simulink model "SIMULINK_FT_SRL_NZS_Tracking_R18b"  (R2018b)
settings: Solver=FixedStepAuto  StartTime=0.0  StopTime=sim_end_time  FixedStep=fixed_step_size  RelTol=1e-3
InitFcn:
  | start_uav_car_10
values from neighbouring files (symbols this model uses):
  a = 1    [start_uav_car_10.m]
  act_end = 2*pi/w1    (= 62.8318530718)    [start_uav_car_10.m]
  b = 1.8    [start_uav_car_10.m]
  battery_threshold = 20    [start_uav_car_10.m]
  bb = 1.2    [start_uav_car_10.m]
  delta_ = [delta_his(2:end,:); delta]    [adp_tracking.m]    (also in start_uav_car_10.m = zeros(N,1))
  draw_gif = false    [start_uav_car_10.m]
  fixed_step_size = 1/30    (= 0.0333333333333)    [start_uav_car_10.m]
  k = 0.2    [start_uav_car_10.m]
  KD_x = 0.000002    (= 2e-06)    [start_uav_car_10.m]
  KD_y = 0.00002    (= 2e-05)    [start_uav_car_10.m]
  kd_z = 0.02    [start_uav_car_10.m]
  KDD_x = 0.0008    [start_uav_car_10.m]
  KDD_y = 0.0008    [start_uav_car_10.m]
  KI_x = 0.000002    (= 2e-06)    [start_uav_car_10.m]
  KI_y = 0.000002    (= 2e-06)    [start_uav_car_10.m]
  ki_z = 0.002    [start_uav_car_10.m]
  KII_x = 0.000000    (= 0)    [start_uav_car_10.m]
  KII_y = 0.000    (= 0)    [start_uav_car_10.m]
  KP_x = 1.5    [start_uav_car_10.m]
  KP_y = 1.5    [start_uav_car_10.m]
  kp_z = 0.7    [start_uav_car_10.m]
  KPP_x = 0.4    [start_uav_car_10.m]
  KPP_y = 0.4    [start_uav_car_10.m]
  lmt = 0.5    [start_uav_car_10.m]
  omega = omega_(i,:)    [adp_tracking.m]    (also in start_uav_car_10.m = 0.3)
  omega_ = [omega_his(2:end,:); omega']    [adp_tracking.m]    (also in start_uav_car_10.m = zeros(N,l))
  R = 200*eye(2)    [adp_tracking.m]    (also in start_uav_car_10.m = 0.7)
  sim_end_time = 300    [start_uav_car_10.m]    (also in trjcar.m = 600)
  UAV_NUM = 1    [start_uav_car_10.m]
  Vel_Switch_1 = 1    [start_uav_car_10.m]
  Vel_Switch_10 = 1    [start_uav_car_10.m]
  Vel_Switch_11 = 1    [start_uav_car_10.m]
  Vel_Switch_12 = 1    [start_uav_car_10.m]
  Vel_Switch_13 = 1    [start_uav_car_10.m]
  Vel_Switch_14 = 1    [start_uav_car_10.m]
  Vel_Switch_15 = 1    [start_uav_car_10.m]
  Vel_Switch_16 = 1    [start_uav_car_10.m]
  Vel_Switch_17 = 1    [start_uav_car_10.m]
  Vel_Switch_18 = 1    [start_uav_car_10.m]
  Vel_Switch_19 = 1    [start_uav_car_10.m]
  Vel_Switch_2 = 1    [start_uav_car_10.m]
  Vel_Switch_20 = 1    [start_uav_car_10.m]
  Vel_Switch_3 = 1    [start_uav_car_10.m]
  Vel_Switch_4 = 1    [start_uav_car_10.m]
  Vel_Switch_5 = 1    [start_uav_car_10.m]
  Vel_Switch_6 = 1    [start_uav_car_10.m]
  Vel_Switch_7 = 1    [start_uav_car_10.m]
  Vel_Switch_8 = 1    [start_uav_car_10.m]
  Vel_Switch_9 = 1    [start_uav_car_10.m]
  W0 = 10*ones(l,1)    [start_uav_car_10.m]
  w1 = 0.1    [start_uav_car_10.m]
  w2 = 30    [start_uav_car_10.m]
  XMAX = 2.8    [start_uav_car_10.m]
  XMIN = -2.8    [start_uav_car_10.m]
  YMAX = 2.2    [start_uav_car_10.m]
  YMIN = -2.2    [start_uav_car_10.m]
  ys = ys_learned - ys_learned(1,:)    [start_uav_car_10.m]
  ys_learned = [-20 -19.9842645881 -19.9722755737 -19.9635643089 -19.9577075469 -19.9543235714 -19.9530686431 -19.9536337356 -19.9557415391 -19.9591437091 -19.9636183405 -19.9689676484 ... (12618 elements, 6309x2)]    [DMP_ref.mat]
  z_d_for_land = 1    [start_uav_car_10.m]
  ZMAX = 2.0    (= 2)    [start_uav_car_10.m]
  ZMIN = 0.7    [start_uav_car_10.m]
undefined symbols (not defined in the file or in its folder): droneyeeUAV2_NUM, droneyeeUAV3_NUM, droneyeeUAV4_NUM, droneyeeUAV5_NUM, uav10num, uav1num, uav2num, uav3num, uav4num, uav5num, uav6num, uav7num, uav8num, uav9num
libraries: simulink x121, aerolibanimutils x1
(part 5 of 11)

== system SIMULINK_FT_SRL_NZS_Tracking_R18b/CMD_car1/CMD6 ==
  "clock " : Inport
  droneyeeUAV_states : Inport  Port=2
  droneyeeUAV_bat : Inport  Port=3
  Bus Selector : BusSelector  OutputSignals=x,y,z
  Constant : Constant  Value=sim_end_time
  Constant1 : Constant  Value=battery_threshold
  Constant2 : Constant  Value=z_d_for_land
  Constant3 : Constant  Value=0
  Constant4 : Constant  Value=UAV_NUM
  MATLAB Function1 : MATLAB Function  TreatAsAtomicUnit=on
  Manual Switch2 : ManualSwitch
  Sine Wave2 : Sin  Amplitude=0.3  Frequency=1.0
  Slider Gain3 : simulink/Math Operations/Slider Gain  gain=1  low=0  high=2
  Subsystem : Subsystem
  x_d : Outport
  y_d : Outport  Port=2
  z_d : Outport  Port=3
  yaw_d : Outport  Port=4
  wires:
  Manual Switch2/1 -> Slider Gain3/1
  Slider Gain3/1 -> yaw_d/1
  Sine Wave2/1 -> Manual Switch2/2
  Constant3/1 -> Manual Switch2/1
  MATLAB Function1/2(y_d_) -> y_d/1
  Constant2/1 -> MATLAB Function1/11(z_d_for_land)
  Subsystem/3(zd) -> MATLAB Function1/3(z_d)
  Constant1/1 -> MATLAB Function1/10(battery_threshold)
  MATLAB Function1/3(z_d_) -> z_d/1
  droneyeeUAV_states/1 -> Subsystem/2(uavstates), Bus Selector/1
  MATLAB Function1/1(x_d_) -> x_d/1
  Constant4/1 -> MATLAB Function1/12(UAV_NUM)
  Constant/1 -> MATLAB Function1/9(sim_time_end)
  Subsystem/1("xd ") -> MATLAB Function1/1(x_d)
  Subsystem/2(yd) -> MATLAB Function1/2(y_d)
  "clock "/1 -> Subsystem/1(clock), MATLAB Function1/4(timestamp)
  droneyeeUAV_bat/1 -> MATLAB Function1/8(battery_status)
  Bus Selector/1 -> MATLAB Function1/5(x)  "<x>"
  Bus Selector/2 -> MATLAB Function1/6(y)  "<y>"
  Bus Selector/3 -> MATLAB Function1/7(z)  "<z>"

== system SIMULINK_FT_SRL_NZS_Tracking_R18b/CMD_car1/CMD7 ==
  "clock " : Inport
  droneyeeUAV_states : Inport  Port=2
  droneyeeUAV_bat : Inport  Port=3
  Bus Selector : BusSelector  OutputSignals=x,y,z
  Constant : Constant  Value=sim_end_time
  Constant1 : Constant  Value=battery_threshold
  Constant2 : Constant  Value=z_d_for_land
  Constant3 : Constant  Value=0
  Constant4 : Constant  Value=UAV_NUM
  MATLAB Function1 : MATLAB Function  TreatAsAtomicUnit=on
  Manual Switch2 : ManualSwitch
  Sine Wave2 : Sin  Amplitude=0.3  Frequency=1.0
  Slider Gain3 : simulink/Math Operations/Slider Gain  gain=1  low=0  high=2
  Subsystem : Subsystem
  Terminator : Terminator
  x_d : Outport
  y_d : Outport  Port=2
  z_d : Outport  Port=3
  yaw_d : Outport  Port=4
  wires:
  Manual Switch2/1 -> Slider Gain3/1
  Slider Gain3/1 -> yaw_d/1
  Sine Wave2/1 -> Manual Switch2/2
  Constant3/1 -> Manual Switch2/1
  Bus Selector/1 -> MATLAB Function1/5(x)  "<x>"
  MATLAB Function1/2(y_d_) -> y_d/1
  Constant2/1 -> MATLAB Function1/11(z_d_for_land)
  Subsystem/3(zd) -> MATLAB Function1/3(z_d)
  Bus Selector/2 -> MATLAB Function1/6(y)  "<y>"
  Constant1/1 -> MATLAB Function1/10(battery_threshold)
  MATLAB Function1/3(z_d_) -> z_d/1
  MATLAB Function1/1(x_d_) -> x_d/1
  Constant4/1 -> MATLAB Function1/12(UAV_NUM)
  Bus Selector/3 -> MATLAB Function1/7(z)  "<z>"
  Constant/1 -> MATLAB Function1/9(sim_time_end)
  Subsystem/1("xd ") -> MATLAB Function1/1(x_d)
  Subsystem/2(yd) -> MATLAB Function1/2(y_d)
  "clock "/1 -> Subsystem/1(clock), MATLAB Function1/4(timestamp)
  droneyeeUAV_bat/1 -> MATLAB Function1/8(battery_status)
  droneyeeUAV_states/1 -> Subsystem/2(uavstates), Bus Selector/1

== system SIMULINK_FT_SRL_NZS_Tracking_R18b/CMD_car1/CMD8 ==
  "clock " : Inport
  droneyeeUAV_states : Inport  Port=2
  droneyeeUAV_bat : Inport  Port=3
  Bus Selector : BusSelector  OutputSignals=x,y,z
  Constant : Constant  Value=sim_end_time
  Constant1 : Constant  Value=battery_threshold
  Constant2 : Constant  Value=z_d_for_land
  Constant3 : Constant  Value=0
  Constant4 : Constant  Value=UAV_NUM
  MATLAB Function1 : MATLAB Function  TreatAsAtomicUnit=on
  Manual Switch2 : ManualSwitch
  Sine Wave2 : Sin  Amplitude=0.3  Frequency=1.0
  Slider Gain3 : simulink/Math Operations/Slider Gain  gain=1  low=0  high=2
  Subsystem : Subsystem
  x_d : Outport
  y_d : Outport  Port=2
  z_d : Outport  Port=3
  yaw_d : Outport  Port=4
  wires:
  Manual Switch2/1 -> Slider Gain3/1
  Slider Gain3/1 -> yaw_d/1
  Sine Wave2/1 -> Manual Switch2/2
  Constant3/1 -> Manual Switch2/1
  MATLAB Function1/2(y_d_) -> y_d/1
  Constant2/1 -> MATLAB Function1/11(z_d_for_land)
  Subsystem/3(zd) -> MATLAB Function1/3(z_d)
  Constant1/1 -> MATLAB Function1/10(battery_threshold)
  MATLAB Function1/3(z_d_) -> z_d/1
  droneyeeUAV_states/1 -> Subsystem/2(uavstates), Bus Selector/1
  MATLAB Function1/1(x_d_) -> x_d/1
  Constant4/1 -> MATLAB Function1/12(UAV_NUM)
  Constant/1 -> MATLAB Function1/9(sim_time_end)
  Subsystem/1("xd ") -> MATLAB Function1/1(x_d)
  Subsystem/2(yd) -> MATLAB Function1/2(y_d)
  "clock "/1 -> Subsystem/1(clock), MATLAB Function1/4(timestamp)
  droneyeeUAV_bat/1 -> MATLAB Function1/8(battery_status)
  Bus Selector/1 -> MATLAB Function1/5(x)  "<x>"
  Bus Selector/2 -> MATLAB Function1/6(y)  "<y>"
  Bus Selector/3 -> MATLAB Function1/7(z)  "<z>"

== system SIMULINK_FT_SRL_NZS_Tracking_R18b/CMD_car1/CMD9 ==
  "clock " : Inport
  droneyeeUAV_states : Inport  Port=2
  droneyeeUAV_bat : Inport  Port=3
  Bus Selector : BusSelector  OutputSignals=x,y,z
  Constant : Constant  Value=sim_end_time
  Constant1 : Constant  Value=battery_threshold
  Constant2 : Constant  Value=z_d_for_land
  Constant3 : Constant  Value=0
  Constant4 : Constant  Value=UAV_NUM
  MATLAB Function1 : MATLAB Function  TreatAsAtomicUnit=on
  Manual Switch2 : ManualSwitch
  Sine Wave2 : Sin  Amplitude=0.3  Frequency=1.0
  Slider Gain3 : simulink/Math Operations/Slider Gain  gain=1  low=0  high=2
  Subsystem : Subsystem
  Terminator : Terminator
  x_d : Outport
  y_d : Outport  Port=2
  z_d : Outport  Port=3
  yaw_d : Outport  Port=4
  wires:
  Manual Switch2/1 -> Slider Gain3/1
  Slider Gain3/1 -> yaw_d/1
  Sine Wave2/1 -> Manual Switch2/2
  Constant3/1 -> Manual Switch2/1
  Bus Selector/1 -> MATLAB Function1/5(x)  "<x>"
  MATLAB Function1/2(y_d_) -> y_d/1
  Constant2/1 -> MATLAB Function1/11(z_d_for_land)
  Subsystem/3(zd) -> MATLAB Function1/3(z_d)
  Bus Selector/2 -> MATLAB Function1/6(y)  "<y>"
  Constant1/1 -> MATLAB Function1/10(battery_threshold)
  MATLAB Function1/3(z_d_) -> z_d/1
  MATLAB Function1/1(x_d_) -> x_d/1
  Constant4/1 -> MATLAB Function1/12(UAV_NUM)
  Bus Selector/3 -> MATLAB Function1/7(z)  "<z>"
  Constant/1 -> MATLAB Function1/9(sim_time_end)
  Subsystem/1("xd ") -> MATLAB Function1/1(x_d)
  Subsystem/2(yd) -> MATLAB Function1/2(y_d)
  "clock "/1 -> Subsystem/1(clock), MATLAB Function1/4(timestamp)
  droneyeeUAV_bat/1 -> MATLAB Function1/8(battery_status)
  droneyeeUAV_states/1 -> Subsystem/2(uavstates), Bus Selector/1

== system SIMULINK_FT_SRL_NZS_Tracking_R18b/control system_UAV/Baseline Controller1 ==
  X_e : Inport
  Y_e : Inport  Port=2
  " Z_e " : Inport  Port=3
  Yaw_e : Inport  Port=4
  " V_x" : Inport  Port=5
  V_y : Inport  Port=6
  "V_z " : Inport  Port=7
  x_d : Inport  Port=8
  y_d : Inport  Port=9
  Z_d : Inport  Port=10
  Yaw_d : Inport  Port=11
  Constant : Constant  Commented=on  Value=omega*R*2
  Demux : Demux  Outputs=2
  Heading controller : Subsystem
  "Height controller " : Subsystem
  MATLAB Function : MATLAB Function  Commented=on  TreatAsAtomicUnit=on
  Position controller : Subsystem
  Saturation1 : Saturate  UpperLimit=lmt  LowerLimit=-lmt
  Saturation2 : Saturate  UpperLimit=lmt  LowerLimit=-lmt
  Scope : Scope  NumInputPorts=6
  input : Scope  NumInputPorts=3
  ux : Outport
  uy : Outport  Port=2
  Z_velocity_d. [-1,1] : Outport  Port=3
  yaw_rate_d [-1,1] : Outport  Port=4
  wires:
  " Z_e "/1 -> Scope/5, "Height controller "/2(Z_e (m))  "z"
  X_e/1 -> Scope/1, Position controller/1(X_e (m))  "x"
  Y_e/1 -> Scope/3, Position controller/2(Y_e (m))  "y"
  Yaw_d/1 -> Heading controller/2(yaw_d. (rad))
  Demux/1 -> ux/1
  Demux/2 -> uy/1
  Constant/1 -> MATLAB Function/2(a)
  Z_d/1 -> Scope/6, "Height controller "/1(Z_d. (m))  "zd"
  x_d/1 -> Scope/2, Position controller/3(X_d (m))  "xd"
  y_d/1 -> Scope/4, Position controller/4(Y_d (m))  "yd"
  Yaw_e/1 -> Heading controller/1(yaw_e (rad))  "yaw"
  "V_z "/1 -> "Height controller "/3(V_z)
  "Height controller "/1(Z_velocity_d (m/s)) -> Saturation2/1
  Saturation1/1 -> input/2, Demux/1
  Position controller/1(uxy) -> Saturation1/1
  Saturation2/1 -> input/1, Z_velocity_d. [-1,1]/1
  Heading controller/1(yaw_rate_d. (rad/s)) -> input/3, yaw_rate_d [-1,1]/1

== system SIMULINK_FT_SRL_NZS_Tracking_R18b/control system_UAV/Baseline Controller10 ==
  X_e : Inport
  Y_e : Inport  Port=2
  " Z_e " : Inport  Port=3
  Yaw_e : Inport  Port=4
  " V_x" : Inport  Port=5
  V_y : Inport  Port=6
  "V_z " : Inport  Port=7
  x_d : Inport  Port=8
  y_d : Inport  Port=9
  Z_d : Inport  Port=10
  Yaw_d : Inport  Port=11
  Demux : Demux  Outputs=2
  Heading controller : Subsystem
  "Height controller " : Subsystem
  Position controller : Subsystem
  Saturation : Saturate  UpperLimit=lmt  LowerLimit=-lmt
  Saturation1 : Saturate  UpperLimit=lmt  LowerLimit=-lmt
  Saturation2 : Saturate  UpperLimit=lmt  LowerLimit=-lmt
  Scope : Scope
  ux : Outport
  uy : Outport  Port=2
  Z_velocity_d. [-1,1] : Outport  Port=3
  yaw_rate_d [-1,1] : Outport  Port=4
  wires:
  X_e/1 -> Position controller/1(X_e (m))
  Y_e/1 -> Position controller/2(Y_e (m))
  Yaw_d/1 -> Heading controller/2(yaw_d. (rad))
  Saturation/1 -> Demux/1
  Demux/1 -> Scope/1, ux/1
  Demux/2 -> uy/1
  x_d/1 -> Position controller/3(X_d (m))
  y_d/1 -> Position controller/4(Y_d (m))
  Yaw_e/1 -> Heading controller/1(yaw_e (rad))  "yaw"
  Position controller/1(uxy) -> Saturation/1
  Z_d/1 -> "Height controller "/1(Z_d. (m))
  " Z_e "/1 -> "Height controller "/2(Z_e (m))
  "Height controller "/1(Z_velocity_d (m/s)) -> Saturation2/1
  "V_z "/1 -> "Height controller "/3(V_z)
  Saturation2/1 -> Z_velocity_d. [-1,1]/1

== system SIMULINK_FT_SRL_NZS_Tracking_R18b/control system_UAV/Baseline Controller2 ==
  X_e : Inport
  Y_e : Inport  Port=2
  " Z_e " : Inport  Port=3
  Yaw_e : Inport  Port=4
  " V_x" : Inport  Port=5
  V_y : Inport  Port=6
  "V_z " : Inport  Port=7
  x_d : Inport  Port=8
  y_d : Inport  Port=9
  Z_d : Inport  Port=10
  Yaw_d : Inport  Port=11
  Constant : Constant  Commented=on  Value=omega*R*2
  Demux : Demux  Outputs=2
  Heading controller : Subsystem
  "Height controller " : Subsystem
  MATLAB Function : MATLAB Function  Commented=on  TreatAsAtomicUnit=on
  Position controller : Subsystem
  Saturation : Saturate  UpperLimit=lmt  LowerLimit=-lmt
  Saturation1 : Saturate  UpperLimit=lmt  LowerLimit=-lmt
  ux : Outport
  uy : Outport  Port=2
  Z_velocity_d. [-1,1] : Outport  Port=3
  yaw_rate_d [-1,1] : Outport  Port=4
  wires:
  Position controller/1(uxy) -> Saturation/1
  Yaw_e/1 -> Heading controller/1(yaw_e (rad))  "yaw"
  y_d/1 -> Position controller/4(Y_d (m))
  x_d/1 -> Position controller/3(X_d (m))
  Constant/1 -> MATLAB Function/2(a)
  Demux/2 -> uy/1
  Demux/1 -> ux/1
  Saturation/1 -> Demux/1
  Yaw_d/1 -> Heading controller/2(yaw_d. (rad))
  Y_e/1 -> Position controller/2(Y_e (m))
  X_e/1 -> Position controller/1(X_e (m))
  Z_d/1 -> "Height controller "/1(Z_d. (m))
  " Z_e "/1 -> "Height controller "/2(Z_e (m))
  "V_z "/1 -> "Height controller "/3(V_z)
  Saturation1/1 -> Z_velocity_d. [-1,1]/1
  "Height controller "/1(Z_velocity_d (m/s)) -> Saturation1/1

== system SIMULINK_FT_SRL_NZS_Tracking_R18b/control system_UAV/Baseline Controller3 ==
  X_e : Inport
  Y_e : Inport  Port=2
  " Z_e " : Inport  Port=3
  Yaw_e : Inport  Port=4
  " V_x" : Inport  Port=5
  V_y : Inport  Port=6
  "V_z " : Inport  Port=7
  x_d : Inport  Port=8
  y_d : Inport  Port=9
  Z_d : Inport  Port=10
  Yaw_d : Inport  Port=11
  Add : Sum
  Add1 : Sum
  Constant : Constant  Commented=on  Value=omega*R*2
  Demux : Demux  Outputs=2
  Demux1 : Demux  Outputs=2
  Heading controller : Subsystem
  "Height controller " : Subsystem
  MATLAB Function : MATLAB Function  Commented=on  TreatAsAtomicUnit=on
  Position controller : Subsystem
  Saturation : Saturate  UpperLimit=lmt  LowerLimit=-lmt
  Saturation1 : Saturate  UpperLimit=lmt  LowerLimit=-lmt
  Saturation2 : Saturate  UpperLimit=lmt  LowerLimit=-lmt
  ux : Outport
  uy : Outport  Port=2
  Z_velocity_d. [-1,1] : Outport  Port=3
  yaw_rate_d [-1,1] : Outport  Port=4
  wires:
  X_e/1 -> Position controller/1(X_e (m))
  Y_e/1 -> Position controller/2(Y_e (m))
  Yaw_d/1 -> Heading controller/2(yaw_d. (rad))
  Saturation/1 -> Demux/1
  Demux/1 -> Add/1
  Demux/2 -> Add1/2
  Constant/1 -> MATLAB Function/2(a)
  x_d/1 -> Position controller/3(X_d (m))
  y_d/1 -> Position controller/4(Y_d (m))
  Yaw_e/1 -> Heading controller/1(yaw_e (rad))  "yaw"
  Position controller/1(uxy) -> Saturation/1
  "Height controller "/1(Z_velocity_d (m/s)) -> Saturation1/1
  " Z_e "/1 -> "Height controller "/2(Z_e (m))
  "V_z "/1 -> "Height controller "/3(V_z)
  Z_d/1 -> "Height controller "/1(Z_d. (m))
  Saturation1/1 -> Z_velocity_d. [-1,1]/1
  Position controller/2(u2xy) -> Saturation2/1
  Demux1/2 -> Add1/1
  Demux1/1 -> Add/2
  Saturation2/1 -> Demux1/1
  Add/1 -> ux/1
  Add1/1 -> uy/1

== system SIMULINK_FT_SRL_NZS_Tracking_R18b/control system_UAV/Baseline Controller4 ==
  X_e : Inport
  Y_e : Inport  Port=2
  " Z_e " : Inport  Port=3
  Yaw_e : Inport  Port=4
  " V_x" : Inport  Port=5
  V_y : Inport  Port=6
  "V_z " : Inport  Port=7
  x_d : Inport  Port=8
  y_d : Inport  Port=9
  Z_d : Inport  Port=10
  Yaw_d : Inport  Port=11
  Constant : Constant  Commented=on  Value=omega*R*2
  Demux : Demux  Outputs=2
  Heading controller : Subsystem
  "Height controller " : Subsystem
  MATLAB Function : MATLAB Function  Commented=on  TreatAsAtomicUnit=on
  Position controller : Subsystem
  Saturation : Saturate  UpperLimit=lmt  LowerLimit=-lmt
  Saturation1 : Saturate  UpperLimit=lmt  LowerLimit=-lmt
  ux : Outport
  uy : Outport  Port=2
  Z_velocity_d. [-1,1] : Outport  Port=3
  yaw_rate_d [-1,1] : Outport  Port=4
  wires:
  Position controller/1(uxy) -> Saturation/1
  Yaw_e/1 -> Heading controller/1(yaw_e (rad))  "yaw"
  y_d/1 -> Position controller/4(Y_d (m))
  x_d/1 -> Position controller/3(X_d (m))
  Constant/1 -> MATLAB Function/2(a)
  Demux/2 -> uy/1
  Demux/1 -> ux/1
  Saturation/1 -> Demux/1
  Yaw_d/1 -> Heading controller/2(yaw_d. (rad))
  Y_e/1 -> Position controller/2(Y_e (m))
  X_e/1 -> Position controller/1(X_e (m))
  Z_d/1 -> "Height controller "/1(Z_d. (m))
  " Z_e "/1 -> "Height controller "/2(Z_e (m))
  Saturation1/1 -> Z_velocity_d. [-1,1]/1
  "Height controller "/1(Z_velocity_d (m/s)) -> Saturation1/1
  "V_z "/1 -> "Height controller "/3(V_z)

== system SIMULINK_FT_SRL_NZS_Tracking_R18b/control system_UAV/Baseline Controller5 ==
  X_e : Inport
  Y_e : Inport  Port=2
  " Z_e " : Inport  Port=3
  Yaw_e : Inport  Port=4
  " V_x" : Inport  Port=5
  V_y : Inport  Port=6
  "V_z " : Inport  Port=7
  x_d : Inport  Port=8
  y_d : Inport  Port=9
  Z_d : Inport  Port=10
  Yaw_d : Inport  Port=11
  Demux : Demux  Outputs=2
  Heading controller : Subsystem
  "Height controller " : Subsystem
  Position controller : Subsystem
  Saturation : Saturate  UpperLimit=lmt  LowerLimit=-lmt
  Saturation1 : Saturate  UpperLimit=lmt  LowerLimit=-lmt
  Saturation2 : Saturate  UpperLimit=lmt  LowerLimit=-lmt
  Scope : Scope
  ux : Outport
  uy : Outport  Port=2
  Z_velocity_d. [-1,1] : Outport  Port=3
  yaw_rate_d [-1,1] : Outport  Port=4
  wires:
  X_e/1 -> Position controller/1(X_e (m))
  Y_e/1 -> Position controller/2(Y_e (m))
  Yaw_d/1 -> Heading controller/2(yaw_d. (rad))
  Saturation/1 -> Demux/1
  Demux/1 -> Scope/1, ux/1
  Demux/2 -> uy/1
  x_d/1 -> Position controller/3(X_d (m))
  y_d/1 -> Position controller/4(Y_d (m))
  Yaw_e/1 -> Heading controller/1(yaw_e (rad))  "yaw"
  Position controller/1(uxy) -> Saturation/1
  Z_d/1 -> "Height controller "/1(Z_d. (m))
  " Z_e "/1 -> "Height controller "/2(Z_e (m))
  "Height controller "/1(Z_velocity_d (m/s)) -> Saturation2/1
  "V_z "/1 -> "Height controller "/3(V_z)
  Saturation2/1 -> Z_velocity_d. [-1,1]/1

== system SIMULINK_FT_SRL_NZS_Tracking_R18b/control system_UAV/Baseline Controller6 ==
  X_e : Inport
  Y_e : Inport  Port=2
  " Z_e " : Inport  Port=3
  Yaw_e : Inport  Port=4
  " V_x" : Inport  Port=5
  V_y : Inport  Port=6
  "V_z " : Inport  Port=7
  x_d : Inport  Port=8
  y_d : Inport  Port=9
  Z_d : Inport  Port=10
  Yaw_d : Inport  Port=11
  Demux : Demux  Outputs=2
  Heading controller : Subsystem
  "Height controller " : Subsystem
  Position controller : Subsystem
  Saturation : Saturate  UpperLimit=lmt  LowerLimit=-lmt
  Saturation1 : Saturate  UpperLimit=lmt  LowerLimit=-lmt
  Saturation2 : Saturate  UpperLimit=lmt  LowerLimit=-lmt
  Scope : Scope
  ux : Outport
  uy : Outport  Port=2
  Z_velocity_d. [-1,1] : Outport  Port=3
  yaw_rate_d [-1,1] : Outport  Port=4
  wires:
  X_e/1 -> Position controller/1(X_e (m))
  Y_e/1 -> Position controller/2(Y_e (m))
  Yaw_d/1 -> Heading controller/2(yaw_d. (rad))
  Saturation/1 -> Demux/1
  Demux/1 -> Scope/1, ux/1
  Demux/2 -> uy/1
  x_d/1 -> Position controller/3(X_d (m))
  y_d/1 -> Position controller/4(Y_d (m))
  Yaw_e/1 -> Heading controller/1(yaw_e (rad))  "yaw"
  Position controller/1(uxy) -> Saturation/1
  Z_d/1 -> "Height controller "/1(Z_d. (m))
  " Z_e "/1 -> "Height controller "/2(Z_e (m))
  "Height controller "/1(Z_velocity_d (m/s)) -> Saturation2/1
  "V_z "/1 -> "Height controller "/3(V_z)
  Saturation2/1 -> Z_velocity_d. [-1,1]/1

== system SIMULINK_FT_SRL_NZS_Tracking_R18b/control system_UAV/Baseline Controller7 ==
  X_e : Inport
  Y_e : Inport  Port=2
  " Z_e " : Inport  Port=3
  Yaw_e : Inport  Port=4
  " V_x" : Inport  Port=5
  V_y : Inport  Port=6
  "V_z " : Inport  Port=7
  x_d : Inport  Port=8
  y_d : Inport  Port=9
  Z_d : Inport  Port=10
  Yaw_d : Inport  Port=11
  Demux : Demux  Outputs=2
  Heading controller : Subsystem
  "Height controller " : Subsystem
  Position controller : Subsystem
  Saturation : Saturate  UpperLimit=lmt  LowerLimit=-lmt
  Saturation1 : Saturate  UpperLimit=lmt  LowerLimit=-lmt
  Saturation2 : Saturate  UpperLimit=lmt  LowerLimit=-lmt
  Scope : Scope
  ux : Outport
  uy : Outport  Port=2
  Z_velocity_d. [-1,1] : Outport  Port=3
  yaw_rate_d [-1,1] : Outport  Port=4
  wires:
  X_e/1 -> Position controller/1(X_e (m))
  Y_e/1 -> Position controller/2(Y_e (m))
  Yaw_d/1 -> Heading controller/2(yaw_d. (rad))
  Saturation/1 -> Demux/1
  Demux/1 -> Scope/1, ux/1
  Demux/2 -> uy/1
  x_d/1 -> Position controller/3(X_d (m))
  y_d/1 -> Position controller/4(Y_d (m))
  Yaw_e/1 -> Heading controller/1(yaw_e (rad))  "yaw"
  Position controller/1(uxy) -> Saturation/1
  Z_d/1 -> "Height controller "/1(Z_d. (m))
  " Z_e "/1 -> "Height controller "/2(Z_e (m))
  "Height controller "/1(Z_velocity_d (m/s)) -> Saturation2/1
  "V_z "/1 -> "Height controller "/3(V_z)
  Saturation2/1 -> Z_velocity_d. [-1,1]/1

== system SIMULINK_FT_SRL_NZS_Tracking_R18b/control system_UAV/Baseline Controller8 ==
  X_e : Inport
  Y_e : Inport  Port=2
  " Z_e " : Inport  Port=3
  Yaw_e : Inport  Port=4
  " V_x" : Inport  Port=5
  V_y : Inport  Port=6
  "V_z " : Inport  Port=7
  x_d : Inport  Port=8
  y_d : Inport  Port=9
  Z_d : Inport  Port=10
  Yaw_d : Inport  Port=11
  Demux : Demux  Outputs=2
  Heading controller : Subsystem
  "Height controller " : Subsystem
  Position controller : Subsystem
  Saturation : Saturate  UpperLimit=lmt  LowerLimit=-lmt
  Saturation1 : Saturate  UpperLimit=lmt  LowerLimit=-lmt
  Saturation2 : Saturate  UpperLimit=lmt  LowerLimit=-lmt
  Scope : Scope
  ux : Outport
  uy : Outport  Port=2
  Z_velocity_d. [-1,1] : Outport  Port=3
  yaw_rate_d [-1,1] : Outport  Port=4
  wires:
  X_e/1 -> Position controller/1(X_e (m))
  Y_e/1 -> Position controller/2(Y_e (m))
  Yaw_d/1 -> Heading controller/2(yaw_d. (rad))
  Saturation/1 -> Demux/1
  Demux/1 -> Scope/1, ux/1
  Demux/2 -> uy/1
  x_d/1 -> Position controller/3(X_d (m))
  y_d/1 -> Position controller/4(Y_d (m))
  Yaw_e/1 -> Heading controller/1(yaw_e (rad))  "yaw"
  Position controller/1(uxy) -> Saturation/1
  Z_d/1 -> "Height controller "/1(Z_d. (m))
  " Z_e "/1 -> "Height controller "/2(Z_e (m))
  "Height controller "/1(Z_velocity_d (m/s)) -> Saturation2/1
  "V_z "/1 -> "Height controller "/3(V_z)
  Saturation2/1 -> Z_velocity_d. [-1,1]/1

== system SIMULINK_FT_SRL_NZS_Tracking_R18b/control system_UAV/Baseline Controller9 ==
  X_e : Inport
  Y_e : Inport  Port=2
  " Z_e " : Inport  Port=3
  Yaw_e : Inport  Port=4
  " V_x" : Inport  Port=5
  V_y : Inport  Port=6
  "V_z " : Inport  Port=7
  x_d : Inport  Port=8
  y_d : Inport  Port=9
  Z_d : Inport  Port=10
  Yaw_d : Inport  Port=11
  Demux : Demux  Outputs=2
  Heading controller : Subsystem
  "Height controller " : Subsystem
  Position controller : Subsystem
  Saturation : Saturate  UpperLimit=lmt  LowerLimit=-lmt
  Saturation1 : Saturate  UpperLimit=lmt  LowerLimit=-lmt
  Saturation2 : Saturate  UpperLimit=lmt  LowerLimit=-lmt
  Scope : Scope
  ux : Outport
  uy : Outport  Port=2
  Z_velocity_d. [-1,1] : Outport  Port=3
  yaw_rate_d [-1,1] : Outport  Port=4
  wires:
  X_e/1 -> Position controller/1(X_e (m))
  Y_e/1 -> Position controller/2(Y_e (m))
  Yaw_d/1 -> Heading controller/2(yaw_d. (rad))
  Saturation/1 -> Demux/1
  Demux/1 -> Scope/1, ux/1
  Demux/2 -> uy/1
  x_d/1 -> Position controller/3(X_d (m))
  y_d/1 -> Position controller/4(Y_d (m))
  Yaw_e/1 -> Heading controller/1(yaw_e (rad))  "yaw"
  Position controller/1(uxy) -> Saturation/1
  Z_d/1 -> "Height controller "/1(Z_d. (m))
  " Z_e "/1 -> "Height controller "/2(Z_e (m))
  "Height controller "/1(Z_velocity_d (m/s)) -> Saturation2/1
  "V_z "/1 -> "Height controller "/3(V_z)
  Saturation2/1 -> Z_velocity_d. [-1,1]/1

== system SIMULINK_FT_SRL_NZS_Tracking_R18b/control system_car1/Baseline Controller1 ==
  X_e : Inport
  Y_e : Inport  Port=2
  " Z_e " : Inport  Port=3
  Yaw_e : Inport  Port=4
  " V_x" : Inport  Port=5
  V_y : Inport  Port=6
  "V_z " : Inport  Port=7
  x_d : Inport  Port=8
  y_d : Inport  Port=9
  Z_d : Inport  Port=10
  Yaw_d : Inport  Port=11
  Constant : Constant  Commented=on  Value=omega*R*2
  Constant1 : Constant  Value=0
  Demux : Demux  Outputs=2
  Heading controller : Subsystem
  "Height controller " : Subsystem
  MATLAB Function : MATLAB Function  Commented=on  TreatAsAtomicUnit=on
  Position controller : Subsystem
  Saturation1 : Saturate  UpperLimit=lmt  LowerLimit=-lmt
  Saturation2 : Saturate  UpperLimit=lmt  LowerLimit=-lmt
  Terminator : Terminator
  ux : Outport
  uy : Outport  Port=2
  Z_velocity_d. [-1,1] : Outport  Port=3
  yaw_rate_d [-1,1] : Outport  Port=4
  wires:
  " Z_e "/1 -> "Height controller "/2(Z_e (m))
  X_e/1 -> Position controller/1(X_e (m))
  Y_e/1 -> Position controller/2(Y_e (m))
  Yaw_d/1 -> Heading controller/2(yaw_d. (rad))
  Demux/1 -> ux/1
  Demux/2 -> uy/1
  Constant/1 -> MATLAB Function/2(a)
  Z_d/1 -> "Height controller "/1(Z_d. (m))
  x_d/1 -> Position controller/3(X_d (m))
  y_d/1 -> Position controller/4(Y_d (m))
  Yaw_e/1 -> Heading controller/1(yaw_e (rad))  "yaw"
  "V_z "/1 -> "Height controller "/3(V_z)
  Heading controller/1(yaw_rate_d. (rad/s)) -> yaw_rate_d [-1,1]/1
  "Height controller "/1(Z_velocity_d (m/s)) -> Saturation2/1
  Saturation1/1 -> Demux/1
  Position controller/1(uxy) -> Saturation1/1
  Constant1/1 -> Z_velocity_d. [-1,1]/1
  Saturation2/1 -> Terminator/1

== system SIMULINK_FT_SRL_NZS_Tracking_R18b/control system_car1/Baseline Controller10 ==
  X_e : Inport
  Y_e : Inport  Port=2
  " Z_e " : Inport  Port=3
  Yaw_e : Inport  Port=4
  " V_x" : Inport  Port=5
  V_y : Inport  Port=6
  "V_z " : Inport  Port=7
  x_d : Inport  Port=8
  y_d : Inport  Port=9
  Z_d : Inport  Port=10
  Yaw_d : Inport  Port=11
  Constant : Constant  Commented=on  Value=omega*R*2
  Constant1 : Constant  Value=0
  Demux : Demux  Outputs=2
  Heading controller : Subsystem
  "Height controller " : Subsystem
  MATLAB Function : MATLAB Function  Commented=on  TreatAsAtomicUnit=on
  Position controller : Subsystem
  Saturation1 : Saturate  UpperLimit=lmt  LowerLimit=-lmt
  Saturation2 : Saturate  UpperLimit=lmt  LowerLimit=-lmt
  Terminator : Terminator
  ux : Outport
  uy : Outport  Port=2
  Z_velocity_d. [-1,1] : Outport  Port=3
  yaw_rate_d [-1,1] : Outport  Port=4
  wires:
  " Z_e "/1 -> "Height controller "/2(Z_e (m))
  X_e/1 -> Position controller/1(X_e (m))
  Y_e/1 -> Position controller/2(Y_e (m))
  Yaw_d/1 -> Heading controller/2(yaw_d. (rad))
  Demux/1 -> ux/1
  Demux/2 -> uy/1
  Constant/1 -> MATLAB Function/2(a)
  Z_d/1 -> "Height controller "/1(Z_d. (m))
  x_d/1 -> Position controller/3(X_d (m))
  y_d/1 -> Position controller/4(Y_d (m))
  Yaw_e/1 -> Heading controller/1(yaw_e (rad))  "yaw"
  "V_z "/1 -> "Height controller "/3(V_z)
  Heading controller/1(yaw_rate_d. (rad/s)) -> yaw_rate_d [-1,1]/1
  "Height controller "/1(Z_velocity_d (m/s)) -> Saturation2/1
  Saturation1/1 -> Demux/1
  Position controller/1(uxy) -> Saturation1/1
  Constant1/1 -> Z_velocity_d. [-1,1]/1
  Saturation2/1 -> Terminator/1

== system SIMULINK_FT_SRL_NZS_Tracking_R18b/control system_car1/Baseline Controller2 ==
  X_e : Inport
  Y_e : Inport  Port=2
  " Z_e " : Inport  Port=3
  Yaw_e : Inport  Port=4
  " V_x" : Inport  Port=5
  V_y : Inport  Port=6
  "V_z " : Inport  Port=7
  x_d : Inport  Port=8
  y_d : Inport  Port=9
  Z_d : Inport  Port=10
  Yaw_d : Inport  Port=11
  Constant : Constant  Commented=on  Value=omega*R*2
  Constant1 : Constant  Value=0
  Demux : Demux  Outputs=2
  Heading controller : Subsystem
  "Height controller " : Subsystem
  MATLAB Function : MATLAB Function  Commented=on  TreatAsAtomicUnit=on
  Position controller : Subsystem
  Saturation1 : Saturate  UpperLimit=lmt  LowerLimit=-lmt
  Saturation2 : Saturate  UpperLimit=lmt  LowerLimit=-lmt
  Terminator : Terminator
  ux : Outport
  uy : Outport  Port=2
  Z_velocity_d. [-1,1] : Outport  Port=3
  yaw_rate_d [-1,1] : Outport  Port=4
  wires:
  " Z_e "/1 -> "Height controller "/2(Z_e (m))
  X_e/1 -> Position controller/1(X_e (m))
  Y_e/1 -> Position controller/2(Y_e (m))
  Yaw_d/1 -> Heading controller/2(yaw_d. (rad))
  Demux/1 -> ux/1
  Demux/2 -> uy/1
  Constant/1 -> MATLAB Function/2(a)
  Z_d/1 -> "Height controller "/1(Z_d. (m))
  x_d/1 -> Position controller/3(X_d (m))
  y_d/1 -> Position controller/4(Y_d (m))
  Yaw_e/1 -> Heading controller/1(yaw_e (rad))  "yaw"
  "V_z "/1 -> "Height controller "/3(V_z)
  Heading controller/1(yaw_rate_d. (rad/s)) -> yaw_rate_d [-1,1]/1
  "Height controller "/1(Z_velocity_d (m/s)) -> Saturation2/1
  Saturation1/1 -> Demux/1
  Position controller/1(uxy) -> Saturation1/1
  Constant1/1 -> Z_velocity_d. [-1,1]/1
  Saturation2/1 -> Terminator/1

== system SIMULINK_FT_SRL_NZS_Tracking_R18b/control system_car1/Baseline Controller3 ==
  X_e : Inport
  Y_e : Inport  Port=2
  " Z_e " : Inport  Port=3
  Yaw_e : Inport  Port=4
  " V_x" : Inport  Port=5
  V_y : Inport  Port=6
  "V_z " : Inport  Port=7
  x_d : Inport  Port=8
  y_d : Inport  Port=9
  Z_d : Inport  Port=10
  Yaw_d : Inport  Port=11
  Constant : Constant  Commented=on  Value=omega*R*2
  Constant1 : Constant  Value=0
  Demux : Demux  Outputs=2
  Heading controller : Subsystem
  "Height controller " : Subsystem
  MATLAB Function : MATLAB Function  Commented=on  TreatAsAtomicUnit=on
  Position controller : Subsystem
  Saturation1 : Saturate  UpperLimit=lmt  LowerLimit=-lmt
  Saturation2 : Saturate  UpperLimit=lmt  LowerLimit=-lmt
  Terminator : Terminator
  ux : Outport
  uy : Outport  Port=2
  Z_velocity_d. [-1,1] : Outport  Port=3
  yaw_rate_d [-1,1] : Outport  Port=4
  wires:
  " Z_e "/1 -> "Height controller "/2(Z_e (m))
  X_e/1 -> Position controller/1(X_e (m))
  Y_e/1 -> Position controller/2(Y_e (m))
  Yaw_d/1 -> Heading controller/2(yaw_d. (rad))
  Demux/1 -> ux/1
  Demux/2 -> uy/1
  Constant/1 -> MATLAB Function/2(a)
  Z_d/1 -> "Height controller "/1(Z_d. (m))
  x_d/1 -> Position controller/3(X_d (m))
  y_d/1 -> Position controller/4(Y_d (m))
  Yaw_e/1 -> Heading controller/1(yaw_e (rad))  "yaw"
  "V_z "/1 -> "Height controller "/3(V_z)
  Heading controller/1(yaw_rate_d. (rad/s)) -> yaw_rate_d [-1,1]/1
  "Height controller "/1(Z_velocity_d (m/s)) -> Saturation2/1
  Saturation1/1 -> Demux/1
  Position controller/1(uxy) -> Saturation1/1
  Constant1/1 -> Z_velocity_d. [-1,1]/1
  Saturation2/1 -> Terminator/1

== system SIMULINK_FT_SRL_NZS_Tracking_R18b/control system_car1/Baseline Controller4 ==
  X_e : Inport
  Y_e : Inport  Port=2
  " Z_e " : Inport  Port=3
  Yaw_e : Inport  Port=4
  " V_x" : Inport  Port=5
  V_y : Inport  Port=6
  "V_z " : Inport  Port=7
  x_d : Inport  Port=8
  y_d : Inport  Port=9
  Z_d : Inport  Port=10
  Yaw_d : Inport  Port=11
  Constant : Constant  Commented=on  Value=omega*R*2
  Constant1 : Constant  Value=0
  Demux : Demux  Outputs=2
  Heading controller : Subsystem
  "Height controller " : Subsystem
  MATLAB Function : MATLAB Function  Commented=on  TreatAsAtomicUnit=on
  Position controller : Subsystem
  Saturation1 : Saturate  UpperLimit=lmt  LowerLimit=-lmt
  Saturation2 : Saturate  UpperLimit=lmt  LowerLimit=-lmt
  Terminator : Terminator
  ux : Outport
  uy : Outport  Port=2
  Z_velocity_d. [-1,1] : Outport  Port=3
  yaw_rate_d [-1,1] : Outport  Port=4
  wires:
  " Z_e "/1 -> "Height controller "/2(Z_e (m))
  X_e/1 -> Position controller/1(X_e (m))
  Y_e/1 -> Position controller/2(Y_e (m))
  Yaw_d/1 -> Heading controller/2(yaw_d. (rad))
  Demux/1 -> ux/1
  Demux/2 -> uy/1
  Constant/1 -> MATLAB Function/2(a)
  Z_d/1 -> "Height controller "/1(Z_d. (m))
  x_d/1 -> Position controller/3(X_d (m))
  y_d/1 -> Position controller/4(Y_d (m))
  Yaw_e/1 -> Heading controller/1(yaw_e (rad))  "yaw"
  "V_z "/1 -> "Height controller "/3(V_z)
  Heading controller/1(yaw_rate_d. (rad/s)) -> yaw_rate_d [-1,1]/1
  "Height controller "/1(Z_velocity_d (m/s)) -> Saturation2/1
  Saturation1/1 -> Demux/1
  Position controller/1(uxy) -> Saturation1/1
  Constant1/1 -> Z_velocity_d. [-1,1]/1
  Saturation2/1 -> Terminator/1

== system SIMULINK_FT_SRL_NZS_Tracking_R18b/control system_car1/Baseline Controller5 ==
  X_e : Inport
  Y_e : Inport  Port=2
  " Z_e " : Inport  Port=3
  Yaw_e : Inport  Port=4
  " V_x" : Inport  Port=5
  V_y : Inport  Port=6
  "V_z " : Inport  Port=7
  x_d : Inport  Port=8
  y_d : Inport  Port=9
  Z_d : Inport  Port=10
  Yaw_d : Inport  Port=11
  Constant : Constant  Commented=on  Value=omega*R*2
  Constant1 : Constant  Value=0
  Demux : Demux  Outputs=2
  Heading controller : Subsystem
  "Height controller " : Subsystem
  MATLAB Function : MATLAB Function  Commented=on  TreatAsAtomicUnit=on
  Position controller : Subsystem
  Saturation1 : Saturate  UpperLimit=lmt  LowerLimit=-lmt
  Saturation2 : Saturate  UpperLimit=lmt  LowerLimit=-lmt
  Terminator : Terminator
  ux : Outport
  uy : Outport  Port=2
  Z_velocity_d. [-1,1] : Outport  Port=3
  yaw_rate_d [-1,1] : Outport  Port=4
  wires:
  " Z_e "/1 -> "Height controller "/2(Z_e (m))
  X_e/1 -> Position controller/1(X_e (m))
  Y_e/1 -> Position controller/2(Y_e (m))
  Yaw_d/1 -> Heading controller/2(yaw_d. (rad))
  Demux/1 -> ux/1
  Demux/2 -> uy/1
  Constant/1 -> MATLAB Function/2(a)
  Z_d/1 -> "Height controller "/1(Z_d. (m))
  x_d/1 -> Position controller/3(X_d (m))
  y_d/1 -> Position controller/4(Y_d (m))
  Yaw_e/1 -> Heading controller/1(yaw_e (rad))  "yaw"
  "V_z "/1 -> "Height controller "/3(V_z)
  Heading controller/1(yaw_rate_d. (rad/s)) -> yaw_rate_d [-1,1]/1
  "Height controller "/1(Z_velocity_d (m/s)) -> Saturation2/1
  Saturation1/1 -> Demux/1
  Position controller/1(uxy) -> Saturation1/1
  Constant1/1 -> Z_velocity_d. [-1,1]/1
  Saturation2/1 -> Terminator/1

== system SIMULINK_FT_SRL_NZS_Tracking_R18b/control system_car1/Baseline Controller6 ==
  X_e : Inport
  Y_e : Inport  Port=2
  " Z_e " : Inport  Port=3
  Yaw_e : Inport  Port=4
  " V_x" : Inport  Port=5
  V_y : Inport  Port=6
  "V_z " : Inport  Port=7
  x_d : Inport  Port=8
  y_d : Inport  Port=9
  Z_d : Inport  Port=10
  Yaw_d : Inport  Port=11
  Constant : Constant  Commented=on  Value=omega*R*2
  Constant1 : Constant  Value=0
  Demux : Demux  Outputs=2
  Heading controller : Subsystem
  "Height controller " : Subsystem
  MATLAB Function : MATLAB Function  Commented=on  TreatAsAtomicUnit=on
  Position controller : Subsystem
  Saturation1 : Saturate  UpperLimit=lmt  LowerLimit=-lmt
  Saturation2 : Saturate  UpperLimit=lmt  LowerLimit=-lmt
  Terminator : Terminator
  ux : Outport
  uy : Outport  Port=2
  Z_velocity_d. [-1,1] : Outport  Port=3
  yaw_rate_d [-1,1] : Outport  Port=4
  wires:
  " Z_e "/1 -> "Height controller "/2(Z_e (m))
  X_e/1 -> Position controller/1(X_e (m))
  Y_e/1 -> Position controller/2(Y_e (m))
  Yaw_d/1 -> Heading controller/2(yaw_d. (rad))
  Demux/1 -> ux/1
  Demux/2 -> uy/1
  Constant/1 -> MATLAB Function/2(a)
  Z_d/1 -> "Height controller "/1(Z_d. (m))
  x_d/1 -> Position controller/3(X_d (m))
  y_d/1 -> Position controller/4(Y_d (m))
  Yaw_e/1 -> Heading controller/1(yaw_e (rad))  "yaw"
  "V_z "/1 -> "Height controller "/3(V_z)
  Heading controller/1(yaw_rate_d. (rad/s)) -> yaw_rate_d [-1,1]/1
  "Height controller "/1(Z_velocity_d (m/s)) -> Saturation2/1
  Saturation1/1 -> Demux/1
  Position controller/1(uxy) -> Saturation1/1
  Constant1/1 -> Z_velocity_d. [-1,1]/1
  Saturation2/1 -> Terminator/1

== system SIMULINK_FT_SRL_NZS_Tracking_R18b/control system_car1/Baseline Controller7 ==
  X_e : Inport
  Y_e : Inport  Port=2
  " Z_e " : Inport  Port=3
  Yaw_e : Inport  Port=4
  " V_x" : Inport  Port=5
  V_y : Inport  Port=6
  "V_z " : Inport  Port=7
  x_d : Inport  Port=8
  y_d : Inport  Port=9
  Z_d : Inport  Port=10
  Yaw_d : Inport  Port=11
  Constant : Constant  Commented=on  Value=omega*R*2
  Constant1 : Constant  Value=0
  Demux : Demux  Outputs=2
  Heading controller : Subsystem
  "Height controller " : Subsystem
  MATLAB Function : MATLAB Function  Commented=on  TreatAsAtomicUnit=on
  Position controller : Subsystem
  Saturation1 : Saturate  UpperLimit=lmt  LowerLimit=-lmt
  Saturation2 : Saturate  UpperLimit=lmt  LowerLimit=-lmt
  Terminator : Terminator
  ux : Outport
  uy : Outport  Port=2
  Z_velocity_d. [-1,1] : Outport  Port=3
  yaw_rate_d [-1,1] : Outport  Port=4
  wires:
  " Z_e "/1 -> "Height controller "/2(Z_e (m))
  X_e/1 -> Position controller/1(X_e (m))
  Y_e/1 -> Position controller/2(Y_e (m))
  Yaw_d/1 -> Heading controller/2(yaw_d. (rad))
  Demux/1 -> ux/1
  Demux/2 -> uy/1
  Constant/1 -> MATLAB Function/2(a)
  Z_d/1 -> "Height controller "/1(Z_d. (m))
  x_d/1 -> Position controller/3(X_d (m))
  y_d/1 -> Position controller/4(Y_d (m))
  Yaw_e/1 -> Heading controller/1(yaw_e (rad))  "yaw"
  "V_z "/1 -> "Height controller "/3(V_z)
  Heading controller/1(yaw_rate_d. (rad/s)) -> yaw_rate_d [-1,1]/1
  "Height controller "/1(Z_velocity_d (m/s)) -> Saturation2/1
  Saturation1/1 -> Demux/1
  Position controller/1(uxy) -> Saturation1/1
  Constant1/1 -> Z_velocity_d. [-1,1]/1
  Saturation2/1 -> Terminator/1

== system SIMULINK_FT_SRL_NZS_Tracking_R18b/control system_car1/Baseline Controller8 ==
  X_e : Inport
  Y_e : Inport  Port=2
  " Z_e " : Inport  Port=3
  Yaw_e : Inport  Port=4
  " V_x" : Inport  Port=5
  V_y : Inport  Port=6
  "V_z " : Inport  Port=7
  x_d : Inport  Port=8
  y_d : Inport  Port=9
  Z_d : Inport  Port=10
  Yaw_d : Inport  Port=11
  Constant : Constant  Commented=on  Value=omega*R*2
  Constant1 : Constant  Value=0
  Demux : Demux  Outputs=2
  Heading controller : Subsystem
  "Height controller " : Subsystem
  MATLAB Function : MATLAB Function  Commented=on  TreatAsAtomicUnit=on
  Position controller : Subsystem
  Saturation1 : Saturate  UpperLimit=lmt  LowerLimit=-lmt
  Saturation2 : Saturate  UpperLimit=lmt  LowerLimit=-lmt
  Terminator : Terminator
  ux : Outport
  uy : Outport  Port=2
  Z_velocity_d. [-1,1] : Outport  Port=3
  yaw_rate_d [-1,1] : Outport  Port=4
  wires:
  " Z_e "/1 -> "Height controller "/2(Z_e (m))
  X_e/1 -> Position controller/1(X_e (m))
  Y_e/1 -> Position controller/2(Y_e (m))
  Yaw_d/1 -> Heading controller/2(yaw_d. (rad))
  Demux/1 -> ux/1
  Demux/2 -> uy/1
  Constant/1 -> MATLAB Function/2(a)
  Z_d/1 -> "Height controller "/1(Z_d. (m))
  x_d/1 -> Position controller/3(X_d (m))
  y_d/1 -> Position controller/4(Y_d (m))
  Yaw_e/1 -> Heading controller/1(yaw_e (rad))  "yaw"
  "V_z "/1 -> "Height controller "/3(V_z)
  Heading controller/1(yaw_rate_d. (rad/s)) -> yaw_rate_d [-1,1]/1
  "Height controller "/1(Z_velocity_d (m/s)) -> Saturation2/1
  Saturation1/1 -> Demux/1
  Position controller/1(uxy) -> Saturation1/1
  Constant1/1 -> Z_velocity_d. [-1,1]/1
  Saturation2/1 -> Terminator/1

== system SIMULINK_FT_SRL_NZS_Tracking_R18b/control system_car1/Baseline Controller9 ==
  X_e : Inport
  Y_e : Inport  Port=2
  " Z_e " : Inport  Port=3
  Yaw_e : Inport  Port=4
  " V_x" : Inport  Port=5
  V_y : Inport  Port=6
  "V_z " : Inport  Port=7
  x_d : Inport  Port=8
  y_d : Inport  Port=9
  Z_d : Inport  Port=10
  Yaw_d : Inport  Port=11
  Constant : Constant  Commented=on  Value=omega*R*2
  Constant1 : Constant  Value=0
  Demux : Demux  Outputs=2
  Heading controller : Subsystem
  "Height controller " : Subsystem
  MATLAB Function : MATLAB Function  Commented=on  TreatAsAtomicUnit=on
  Position controller : Subsystem
  Saturation1 : Saturate  UpperLimit=lmt  LowerLimit=-lmt
  Saturation2 : Saturate  UpperLimit=lmt  LowerLimit=-lmt
  Terminator : Terminator
  ux : Outport
  uy : Outport  Port=2
  Z_velocity_d. [-1,1] : Outport  Port=3
  yaw_rate_d [-1,1] : Outport  Port=4
  wires:
  " Z_e "/1 -> "Height controller "/2(Z_e (m))
  X_e/1 -> Position controller/1(X_e (m))
  Y_e/1 -> Position controller/2(Y_e (m))
  Yaw_d/1 -> Heading controller/2(yaw_d. (rad))
  Demux/1 -> ux/1
  Demux/2 -> uy/1
  Constant/1 -> MATLAB Function/2(a)
  Z_d/1 -> "Height controller "/1(Z_d. (m))
  x_d/1 -> Position controller/3(X_d (m))
  y_d/1 -> Position controller/4(Y_d (m))
  Yaw_e/1 -> Heading controller/1(yaw_e (rad))  "yaw"
  "V_z "/1 -> "Height controller "/3(V_z)
  Heading controller/1(yaw_rate_d. (rad/s)) -> yaw_rate_d [-1,1]/1
  "Height controller "/1(Z_velocity_d (m/s)) -> Saturation2/1
  Saturation1/1 -> Demux/1
  Position controller/1(uxy) -> Saturation1/1
  Constant1/1 -> Z_velocity_d. [-1,1]/1
  Saturation2/1 -> Terminator/1

== system SIMULINK_FT_SRL_NZS_Tracking_R18b/plot/Subsystem ==
  Constant : Constant  Value=fixed_step_size
  Constant1 : Constant  Value=XMIN
  Constant10 : Constant  Value=b
  Constant11 : Constant  Value=k
  Constant12 : Constant  Value=bb
  Constant13 : Constant  Value=w1
  Constant14 : Constant  Value=w2
  Constant2 : Constant  Value=XMAX
  Constant3 : Constant  Value=YMIN
  Constant4 : Constant  Value=YMAX
  Constant5 : Constant  Value=ZMIN
  Constant6 : Constant  Value=ZMAX
  Constant7 : Constant  Value=draw_gif
  Constant8 : Constant  Value=act_end
  Constant9 : Constant  Value=a
  step_time : Outport
  act_end : Outport  Port=2
  x_min : Outport  Port=3
  x_max : Outport  Port=4
  y_min : Outport  Port=5
  y_max : Outport  Port=6
  z_min : Outport  Port=7
  z_max : Outport  Port=8
  a : Outport  Port=9
  b : Outport  Port=10
  k : Outport  Port=11
  bb : Outport  Port=12
  w1 : Outport  Port=13
  w2 : Outport  Port=14
  draw_gif : Outport  Port=15
  wires:
  Constant/1 -> step_time/1
  Constant1/1 -> x_min/1
  Constant2/1 -> x_max/1
  Constant3/1 -> y_min/1
  Constant4/1 -> y_max/1
  Constant7/1 -> draw_gif/1
  Constant6/1 -> z_max/1
  Constant5/1 -> z_min/1
  Constant13/1 -> w1/1
  Constant10/1 -> b/1
  Constant9/1 -> a/1
  Constant14/1 -> w2/1
  Constant11/1 -> k/1
  Constant8/1 -> act_end/1
  Constant12/1 -> bb/1

== system SIMULINK_FT_SRL_NZS_Tracking_R18b/send_ctrl_signal_UAV/Send Command 1 ==
  pos : Inport
  u : Inport  Port=2
  Bus Selector : BusSelector  OutputSignals=droneyeeUAV1_states.x,droneyeeUAV1_states.y  OutputAsBus=on
  Bus Selector1 : BusSelector  OutputSignals=uav1.u_vx,uav1.u_vy,uav1.u_vz,uav1.u_rate_roll,uav1.u_rate_pitch,uav1.u_rate_yaw
  Clock : Clock
  Compare To Constant : simulink/Logic and Bit Operations/Compare To Constant  relop=>=  const=0.1  OutDataTypeStr=boolean
  Constant : Constant  Value=sim_end_time
  Constant1 : Constant  Value=0
  Constant2 : Constant  Value=uav1num
  Constant3 : Constant  Value=Vel_Switch_1
  Constant4 : Constant  Value=0
  Constant5 : Constant  Value=0
  K : Gain
  K1 : Gain
  K2 : Gain
  Logical Operator : Logic  Inputs=3  AllPortsSameDT=off  OutDataTypeStr=boolean
  Mux : Mux  Inputs=8
  Mux1 : Mux  Inputs=5
  Subsystem : Subsystem
  Sum : Sum  Inputs=|-+
  Switch{1..3,6,12} (5 alike) : Switch  Criteria=u2 > Threshold  Threshold=0.001
  Switch4 : Switch  Criteria=u2 > Threshold
  Switch5 : Switch  Criteria=u2 > Threshold
  uav1 : Constant  Value=0
  tag scope: copterSend1=global, mode1=global, sim_CopterSend1=global
  wires:
  Constant1/1 -> Switch3/3, Switch2/3, Switch1/3, Switch12/3
  K1/1 -> Mux1/5, Mux/7
  Switch1/1 -> K/1
  Bus Selector1/2 -> Switch1/1  "<u_vy>"
  Switch2/1 -> K2/1
  Bus Selector1/3 -> Switch2/1  "<u_vz>"
  Switch3/1 -> K1/1
  Logical Operator/1 -> Switch1/2, Switch12/2, Switch2/2, Switch3/2
  K2/1 -> Mux1/4, Mux/4
  Clock/1 -> Sum/1
  Constant/1 -> Sum/2
  Sum/1 -> Compare To Constant/1
  Compare To Constant/1 -> Logical Operator/2
  pos/1 -> Bus Selector/1
  Bus Selector/1 -> Subsystem/1(In1)
  u/1 -> Bus Selector1/1
  Bus Selector1/1 -> Switch12/1  "<u_vx>"
  Bus Selector1/6 -> Switch3/1  "<u_rate_yaw>"
  Bus Selector1/4 -> Mux/5  "<u_rate_roll>"
  Bus Selector1/5 -> Mux/6  "<u_rate_pitch>"
  Constant2/1 -> Mux/1
  Constant3/1 -> Logical Operator/3
  Switch12/1 -> Mux1/2, Mux/2
  K/1 -> Mux1/3, Mux/3
  Switch6/1 -> Mux/8
  Subsystem/1(Out1) -> Logical Operator/1
  Constant4/1 -> Mux1/1
  Switch4/1 -> [sim_CopterSend1]
  Mux1/1 -> Switch4/3
  Mux/1 -> Switch5/1
  Switch5/1 -> [copterSend1]
  [sim_flag] -> Switch5/2, Switch4/2
  Constant5/1 -> [mode1]
  uav1/1 -> Switch6/3
  [mode1] -> Switch6/2, Switch6/1

== system SIMULINK_FT_SRL_NZS_Tracking_R18b/send_ctrl_signal_UAV/Send Command 10 ==
  pos : Inport
  u : Inport  Port=2
  Bus Selector : BusSelector  OutputSignals=x,y  OutputAsBus=on
  Bus Selector1 : BusSelector  OutputSignals=u_vx,u_vy,u_vz,u_rate_roll,u_rate_pitch,u_rate_yaw
  Clock : Clock
  Compare To Constant : simulink/Logic and Bit Operations/Compare To Constant  relop=>=  const=0.1  OutDataTypeStr=boolean
  Constant : Constant  Value=sim_end_time
  Constant1 : Constant  Value=0
  Constant2 : Constant  Value=uav10num
  Constant3 : Constant  Value=Vel_Switch_10
  Constant4 : Constant  Value=0
  K : Gain
  K1 : Gain
  K2 : Gain
  Logical Operator : Logic  Inputs=3  AllPortsSameDT=off  OutDataTypeStr=boolean
  Mux : Mux  Inputs=8
  Mux1 : Mux  Inputs=5
  Subsystem : Subsystem
  Sum : Sum  Inputs=|-+
  Switch{1..3,6,12} (5 alike) : Switch  Criteria=u2 > Threshold  Threshold=0.001
  Switch4 : Switch  Criteria=u2 > Threshold
  Switch5 : Switch  Criteria=u2 > Threshold
  uav10 : Constant
  tag scope: copterSend10=global, sim_CopterSend10=global
  wires:
  Constant1/1 -> Switch3/3, Switch2/3, Switch1/3, Switch12/3
  K1/1 -> Mux1/5, Mux/7
  Switch1/1 -> K/1
  Bus Selector1/2 -> Switch1/1  "<u_vy>"
  Switch2/1 -> K2/1
  Bus Selector1/3 -> Switch2/1  "<u_vz>"
  Switch3/1 -> K1/1
  Logical Operator/1 -> Switch1/2, Switch12/2, Switch2/2, Switch3/2
  K2/1 -> Mux1/4, Mux/4
  Clock/1 -> Sum/1
  Constant/1 -> Sum/2
  Sum/1 -> Compare To Constant/1
  Compare To Constant/1 -> Logical Operator/2
  pos/1 -> Bus Selector/1
  Bus Selector/1 -> Subsystem/1(In1)
  u/1 -> Bus Selector1/1
  Bus Selector1/1 -> Switch12/1  "<u_vx>"
  Bus Selector1/6 -> Switch3/1  "<u_rate_yaw>"
  Bus Selector1/4 -> Mux/5  "<u_rate_roll>"
  Bus Selector1/5 -> Mux/6  "<u_rate_pitch>"
  Constant2/1 -> Mux/1
  Constant3/1 -> Logical Operator/3
  Switch12/1 -> Mux1/2, Mux/2
  K/1 -> Mux1/3, Mux/3
  Switch6/1 -> Mux/8
  Subsystem/1(Out1) -> Logical Operator/1
  Constant4/1 -> Mux1/1
  Switch4/1 -> [sim_CopterSend10]
  Mux1/1 -> Switch4/3
  Mux/1 -> Switch5/1
  Switch5/1 -> [copterSend10]
  [sim_flag] -> Switch5/2, Switch4/2
  uav10/1 -> Switch6/3
  [mode1] -> Switch6/2, Switch6/1

== system SIMULINK_FT_SRL_NZS_Tracking_R18b/send_ctrl_signal_UAV/Send Command 2 ==
  pos : Inport
  u : Inport  Port=2
  Bus Selector : BusSelector  OutputSignals=droneyeeUAV2_states.x,droneyeeUAV2_states.y  OutputAsBus=on
  Bus Selector1 : BusSelector  OutputSignals=uav2.u_vx,uav2.u_vy,uav2.u_vz,uav2.u_rate_roll,uav2.u_rate_pitch,uav2.u_rate_yaw
  Clock : Clock
  Compare To Constant : simulink/Logic and Bit Operations/Compare To Constant  relop=>=  const=0.1  OutDataTypeStr=boolean
  Constant : Constant  Value=sim_end_time
  Constant1 : Constant  Value=0
  Constant2 : Constant  Value=droneyeeUAV2_NUM
  Constant3 : Constant  Value=Vel_Switch_2
  Constant4 : Constant  Value=0
  K : Gain
  K1 : Gain
  K2 : Gain
  Logical Operator : Logic  Inputs=3  AllPortsSameDT=off  OutDataTypeStr=boolean
  Mux : Mux  Inputs=8
  Mux1 : Mux  Inputs=5
  Subsystem : Subsystem
  Sum : Sum  Inputs=|-+
  Switch{1..3,6,12} (5 alike) : Switch  Criteria=u2 > Threshold  Threshold=0.001
  Switch4 : Switch  Criteria=u2 > Threshold
  Switch5 : Switch  Criteria=u2 > Threshold
  uav2 : Constant
  tag scope: copterSend2=global, sim_CopterSend2=global
  wires:
  Constant1/1 -> Switch3/3, Switch2/3, Switch1/3, Switch12/3
  Switch1/1 -> K/1
  Bus Selector1/2 -> Switch1/1  "<u_vy>"
  Switch2/1 -> K2/1
  Bus Selector1/3 -> Switch2/1  "<u_vz>"
  Switch3/1 -> K1/1
  Logical Operator/1 -> Switch1/2, Switch12/2, Switch2/2, Switch3/2
  Clock/1 -> Sum/1
  Constant/1 -> Sum/2
  Sum/1 -> Compare To Constant/1
  Compare To Constant/1 -> Logical Operator/2
  pos/1 -> Bus Selector/1
  Bus Selector/1 -> Subsystem/1(In1)
  u/1 -> Bus Selector1/1
  Bus Selector1/1 -> Switch12/1  "<u_vx>"
  Bus Selector1/6 -> Switch3/1  "<u_rate_yaw>"
  Bus Selector1/4 -> Mux/5  "<u_rate_roll>"
  Bus Selector1/5 -> Mux/6  "<u_rate_pitch>"
  Constant2/1 -> Mux/1
  Constant3/1 -> Logical Operator/3
  Switch6/1 -> Mux/8
  Subsystem/1(Out1) -> Logical Operator/1
  Switch4/1 -> [sim_CopterSend2]
  [sim_flag] -> Switch5/2, Switch4/2
  Switch5/1 -> [copterSend2]
  Mux/1 -> Switch5/1
  Mux1/1 -> Switch4/3
  K/1 -> Mux1/3, Mux/3
  K1/1 -> Mux1/5, Mux/7
  K2/1 -> Mux1/4, Mux/4
  Switch12/1 -> Mux1/2, Mux/2
  Constant4/1 -> Mux1/1
  uav2/1 -> Switch6/3
  [mode1] -> Switch6/2, Switch6/1
